simulink model "Par6TestDelay"  (R2018a)
settings: Solver=VariableStepAuto  StartTime=0.0  StopTime=10  RelTol=1e-3
settings Model: Creator=wangluo  LastModifiedBy=wangluo

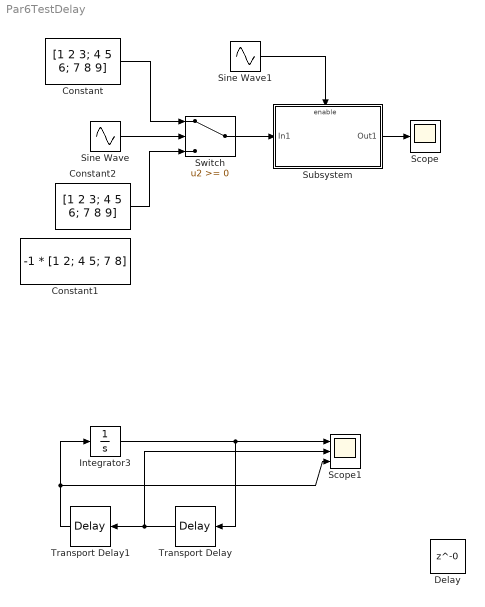
== system Par6TestDelay ==
  Constant : Constant  Value=[1 2 3; 4 5 6; 7 8 9]
  Constant1 : Constant  Value=-1 * [1 2; 4 5; 7 8]
  Constant2 : Constant  Value=[1 2 3; 4 5 6; 7 8 9]
  Delay : Delay  DelayLength=0  InitialCondition=0
  Integrator3 : Integrator  InitialCondition=-6
  Scope : Scope
  Scope1 : Scope  NumInputPorts=3
  Sine Wave : Sin  SampleTime=0
  Sine Wave1 : Sin  SampleTime=0
  Subsystem : Subsystem
  Switch : Switch
  Transport Delay : TransportDelay
  Transport Delay1 : TransportDelay
  wires:
  Sine Wave/1 -> Switch/2
  Constant/1 -> Switch/1
  Constant2/1 -> Switch/3
  Switch/1 -> Subsystem/1(In1)
  Subsystem/1(Out1) -> Scope/1
  Sine Wave1/1 -> Subsystem/Enable
  Integrator3/1 -> Transport Delay/1, Scope1/1
  Transport Delay/1 -> Transport Delay1/1, Scope1/2
  Transport Delay1/1 -> Integrator3/1, Scope1/3

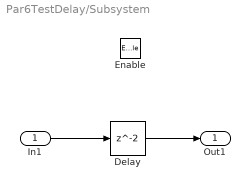
== system Par6TestDelay/Subsystem ==
  In1 : Inport
  Enable : EnablePort
  Delay : Delay  InitialCondition=0
  Out1 : Outport
  wires:
  In1/1 -> Delay/1
  Delay/1 -> Out1/1
